simulink model "LKAS_AutoSave_DF_20220408_1006_SW62"  (R2018b)
settings: Solver=FixedStepDiscrete  StartTime=0.0  StopTime=10.0  FixedStep=0.01  RelTol=1e-3
undefined symbols (not defined in the file): LKA_CarWidth, LKA_SampleTime, LKA_StrRatio_C, LKA_Veh2CamL_C, LKA_Veh2CamW_C, LKA_WhlBaseL_C, LL_CompHdAg_C, LL_CompSWA_C, LL_CrvtPrvwT_C, LL_DesDvt_C, LL_DvtComp_C, LL_DvtPrvwT_C, LL_DvtSpdDet_vDvtSpdMin_C, LL_HandsOff_ExitTime, LL_HandsOff_TextTime, LL_HandsOff_WarnTime, LL_HdAgExT_C, LL_HdAgPrvwT_C, LL_LAccMax_C, LL_LAccRMax_C, LL_LDW_EarliestWarnLine_C, LL_LDW_LatestWarnLine_C, LL_LDWS_SUPPRESS_HEADING, LL_LFClb_TFC_FfCtlRatio_C, LL_LFClb_TFC_KdBalance_C, LL_LFClb_TFC_KdMaxSWA_C, LL_LFClb_TFC_KdV1_C, LL_LFClb_TFC_KdV2_C, LL_LFClb_TFC_KdVehSpdLwr_C, LL_LFClb_TFC_KdVehSpdUpr_C, LL_LFClb_TFC_Ki_C, LL_LFClb_TFC_KiMaxSWA_C, LL_LFClb_TFC_Kp_C, LL_LFClb_TFC_KpKlat_C, LL_LFClb_TFC_KpV1_C, LL_LFClb_TFC_KpV2_C, LL_LFClb_TFC_KpVehSpdLwr_C, LL_LFClb_TFC_KpVehSpdUpr_C, LL_LFClb_TFC_PrvwT_C, LL_LKA_EarliestWarnLine_C, LL_LKA_LatestWarnLine_C, LL_LKAExPrcs_ExitC0Dvt, LL_LKAExPrcs_ExitC0Swt, LL_LKAExPrcs_tiExitDelayTime3, LL_LKAExPrcs_tiExitTime1, LL_LKAExPrcs_tiExitTime2, LL_LKAExPrcs_tiExitTime3, LL_LKAS_OUT_OF_CONTROL_LAT_VEL, LL_LKAS_OUT_OF_CONTROL_TTLC, LL_LKASWASyn_M0, LL_LKASWASyn_M1, LL_LKASWASyn_M2, LL_LKASWASyn_M3D, LL_LKASWASyn_M3K_DT, LL_LKASWASyn_M3K_MSD, LL_LKASWASyn_M4K, LL_LKASWASyn_SWAaddMax, LL_LKASWASyn_T2, LL_LKASWASyn_tiTrqSwaRtTime, LL_LKASWASyn_tiTrqSwaTime ... (+47)
libraries: simulink x234, canmsglib x6, dspstat3 x3, simulink_extras x1
(part 1 of 16)
settings Model: Creator=hejr  LastModifiedBy=hejr
settings OptimizationCC: BlockReduction=off  DefaultParameterBehavior=Inlined  UseDivisionForNetSlopeComputation=on  UseFloatMulNetSlope=on  DefaultUnderspecifiedDataType=single  UseSpecifiedMinMax=on  InlineInvariantSignals=on  PassReuseOutputArgsAs=Individual arguments  ZeroExternalMemoryAtStartup=off  ZeroInternalMemoryAtStartup=off  NoFixptDivByZeroProtection=on  EfficientFloat2IntCast=on  LifeSpan=inf  OptimizeBlockOrder=speed  DifferentSizesBufferReuse=on
settings DebuggingCC: SignalInfNanChecking=error  ReadBeforeWriteMsg=EnableAllAsError  WriteAfterWriteMsg=EnableAllAsError  WriteAfterReadMsg=EnableAllAsError  IntegerOverflowMsg=error  ParameterTunabilityLossMsg=error  UniqueDataStoreMsg=error  AssertControl=DisableAll  NonBusSignalsTreatedAsBus=error  SFInvalidInputDataAccessInChartInitDiag=error  SFTransitionOutsideNaturalParentDiag=error  SFUnreachableExecutionPathDiag=error  SFUndirectedBroadcastEventsDiag=error  IntegerSaturationMsg=error
settings HardwareCC: ProdLongLongMode=on
settings ModelReferenceCC: UpdateModelReferenceTargets=IfOutOfDate
settings SFSimCC: SFSimEcho=off  CompileTimeRecursionLimit=0  EnableRuntimeRecursion=off  MATLABDynamicMemAlloc=off
settings RTWCC: SystemTargetFile=autosar.tlc  GenCodeOnly=on  TemplateMakefile=ert_default_tmf  Description=AUTOSAR  GenerateReport=on  BuildConfiguration=Faster Runs  IncludeHyperlinkInReport=on  LaunchReport=on  GenerateTraceInfo=on  GenerateTraceReport=on  GenerateTraceReportSl=on  GenerateTraceReportSf=on  GenerateTraceReportEml=on  GenerateCodeMetricsReport=on  GenerateCodeReplacementReport=on
settings CodeAppCC: ForceParamTrailComments=on  IgnoreCustomStorageClasses=off  OperatorAnnotations=on  SimulinkDataObjDesc=on  SFDataObjDesc=on  MATLABFcnDesc=on  InsertBlockDesc=on  StateflowObjectComments=on  MATLABSourceComments=on  EnableCustomComments=on  ReqsInCode=on
settings STFCustomTargetCC: TargetLangStandard=C99 (ISO)  MultiwordLength=256  ParMdlRefBuildCompliant=on  CompOptLevelCompliant=on  IncludeMdlTerminateFcn=off  CombineOutputUpdateFcns=on  CombineSignalStateStructs=on  SuppressErrorStatus=on  ERTCustomFileBanners=on  SupportNonFinite=off  SupportComplex=off  SupportContinuousTime=off  SupportNonInlinedSFcns=off  RemoveResetFunc=on  ParenthesesLevel=Maximum  CastingMode=Standards  MATLABClassNameForMDSCustomization=Simulink.SoftwareTarget.ERTCustomization  AutosarCompliant=on  UseToolchainInfoCompliant=on  LookupTableObjectStructAxisOrder=2,1,3,4,...  LUTObjectStructOrderEvenSpacing=Size,Table,Breakpoints  SystemTargetFile=autosar.tlc
settings ERTTargetCC: TargetLangStandard=C99 (ISO)  ConcurrentExecutionCompliant=off  IncludeMdlTerminateFcn=off  CombineSignalStateStructs=on  SuppressErrorStatus=on  SupportNonFinite=off  SupportComplex=off  ParenthesesLevel=Maximum  CastingMode=Standards  ModelStepFunctionPrototypeControlCompliant=off  CPPClassGenCompliant=off  AutosarCompliant=on  LookupTableObjectStructAxisOrder=2,1,3,4,...  LUTObjectStructOrderEvenSpacing=Size,Table,Breakpoints  GenerateASAP2=on  InlinedParameterPlacement=NonHierarchical  ERTCustomFileTemplate=example_file_process.tlc  EnableSignedLeftShifts=off  EnableSignedRightShifts=off

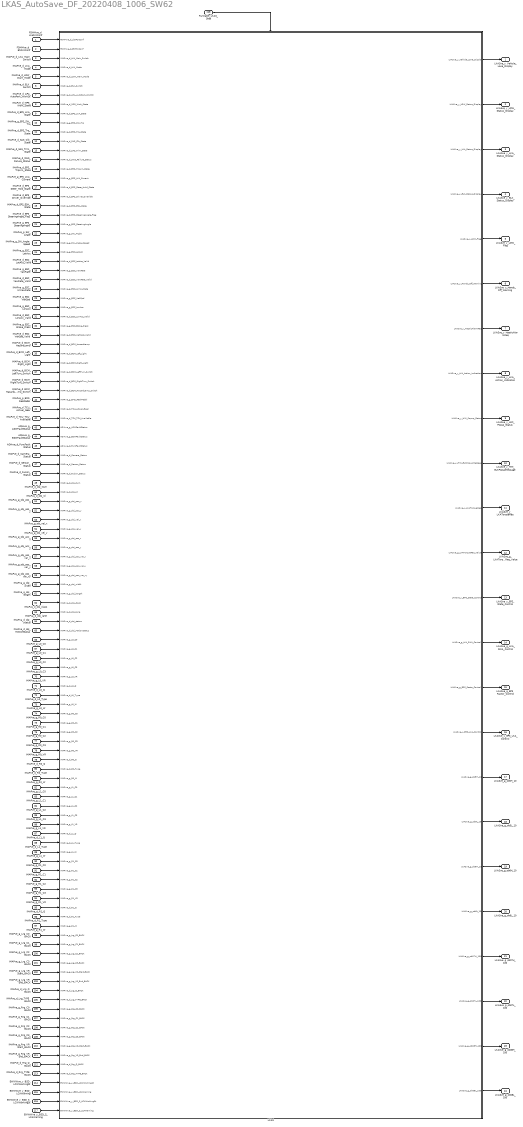
== system LKAS_AutoSave_DF_20220408_1006_SW62 ==
  FDMMve_d_LkaFcnConf : Inport  OutDataTypeStr=UInt16  PortDimensions=1
  FDMMve_d_ElkFcnConf : Inport  Port=2  OutDataTypeStr=UInt16  PortDimensions=1
  IMAPve_d_LKA_Main_Switch : Inport  Port=3  OutDataTypeStr=UInt16  PortDimensions=1
  IMAPve_d_LKA_Mode : Inport  Port=4  OutDataTypeStr=UInt16  PortDimensions=1
  IMAPve_d_LDW_Warn_Mode : Inport  Port=5  OutDataTypeStr=UInt16  PortDimensions=1
  IMAPve_d_ELK_Switch : Inport  Port=6  OutDataTypeStr=UInt16  PortDimensions=1
  IMAPve_d_APA_AutoPark_WorkSt : Inport  Port=7  OutDataTypeStr=UInt16  PortDimensions=1
  IMAPve_d_MP5_Work_State : Inport  Port=8  OutDataTypeStr=UInt16  PortDimensions=1
  IMAPve_d_EPS_LKA_State : Inport  Port=9  OutDataTypeStr=UInt16  PortDimensions=1
  IMAPve_g_EPS_SW_Trq : Inport  Port=10  OutDataTypeStr=T_M_Nm_Float32  PortDimensions=1
  IMAPve_d_EPS_Trq_State : Inport  Port=11  OutDataTypeStr=UInt16  PortDimensions=1
  IMAPve_d_SAS_Clb_State : Inport  Port=12  OutDataTypeStr=UInt16  PortDimensions=1
  IMAPve_d_SAS_Trim_State : Inport  Port=13  OutDataTypeStr=UInt16  PortDimensions=1
  IMAPve_d_SWS_Failure_Status : Inport  Port=14  OutDataTypeStr=UInt16  PortDimensions=1
  IMAPve_d_EPS_TrqLim_State : Inport  Port=15  OutDataTypeStr=UInt16  PortDimensions=1
  IMAPve_g_EPS_LKA_Current : Inport  Port=16  OutDataTypeStr=T_M_Nm_Float32  PortDimensions=1
  IMAPve_d_EPS_Steer_Hold_State : Inport  Port=17  OutDataTypeStr=UInt16  PortDimensions=1
  IMAPve_d_EPS_Driver_Override : Inport  Port=18  OutDataTypeStr=UInt16  PortDimensions=1
  IMAPve_d_EPS_ESA_State : Inport  Port=19  OutDataTypeStr=UInt16  PortDimensions=1
  IMAPve_d_EPS_SteeringAngle_Flag : Inport  Port=20  OutDataTypeStr=UInt16  PortDimensions=1
  IMAPve_g_EPS_SteeringAngle : Inport  Port=21  OutDataTypeStr=T_M_Nm_Float32  PortDimensions=1
  IMAPve_g_SW_Angle : Inport  Port=22  OutDataTypeStr=T_M_Nm_Float32  PortDimensions=1
  IMAPve_g_SW_Angle_Speed : Inport  Port=23  OutDataTypeStr=T_M_Nm_Float32  PortDimensions=1
  IMAPve_g_ESC_LatAcc : Inport  Port=24  OutDataTypeStr=T_M_Nm_Float32  PortDimensions=1
  IMAPve_d_ESC_LatAcc_Valid : Inport  Port=25  OutDataTypeStr=UInt16  PortDimensions=1
  IMAPve_g_ESC_YawRate : Inport  Port=26  OutDataTypeStr=T_M_Nm_Float32  PortDimensions=1
  IMAPve_d_ESC_YawRate_Valid : Inport  Port=27  OutDataTypeStr=UInt16  PortDimensions=1
  IMAPve_g_ESC_UnYawRate : Inport  Port=28  OutDataTypeStr=T_M_Nm_Float32  PortDimensions=1
  IMAPve_g_ESC_VehSpd : Inport  Port=29  OutDataTypeStr=T_M_Nm_Float32  PortDimensions=1
  IMAPve_g_ESC_LonAcc : Inport  Port=30  OutDataTypeStr=T_M_Nm_Float32  PortDimensions=1
  IMAPve_d_ESC_LonAcc_Valid : Inport  Port=31  OutDataTypeStr=UInt16  PortDimensions=1
  IMAPve_g_ESC_Brake_Press : Inport  Port=32  OutDataTypeStr=T_M_Nm_Float32  PortDimensions=1
  IMAPve_d_ESC_VehSpd_Valid : Inport  Port=33  OutDataTypeStr=UInt16  PortDimensions=1
  IMAPve_d_BCM_HazardLamp : Inport  Port=34  OutDataTypeStr=UInt16  PortDimensions=1
  IMAPve_d_BCM_Left_Light : Inport  Port=35  OutDataTypeStr=UInt16  PortDimensions=1
  IMAPve_d_BCM_Right_Light : Inport  Port=36  OutDataTypeStr=UInt16  PortDimensions=1
  IMAPve_d_BCM_LeftTurn_Switch : Inport  Port=37  OutDataTypeStr=UInt16  PortDimensions=1
  IMAPve_d_BCM_RightTurn_Switch : Inport  Port=38  OutDataTypeStr=UInt16  PortDimensions=1
  IMAPve_d_BCM_HazardLamp_Switch : Inport  Port=39  OutDataTypeStr=UInt16  PortDimensions=1
  IMAPve_g_EMS_RealPedal : Inport  Port=40  OutDataTypeStr=T_M_Nm_Float32  PortDimensions=1
  IMAPve_d_TCU_Actual_Gear : Inport  Port=41  OutDataTypeStr=UInt16  PortDimensions=1
  IMAPve_d_TCU_TCU_Available : Inport  Port=42  OutDataTypeStr=UInt16  PortDimensions=1
  ADIAve_g_ASWFaultStatus : Inport  Port=43  OutDataTypeStr=T_M_Nm_Float32  PortDimensions=1
  ADIAve_g_BSWFaultStatus : Inport  Port=44  OutDataTypeStr=T_M_Nm_Float32  PortDimensions=1
  ADIAve_d_FuncFaultStatus : Inport  Port=45  OutDataTypeStr=UInt16  PortDimensions=1
  IMAPve_d_Camera_Status : Inport  Port=46  OutDataTypeStr=UInt16  PortDimensions=1
  IMAPve_d_Sensor_Status : Inport  Port=47  OutDataTypeStr=UInt16  PortDimensions=1
  IMAPve_d_Fusion_Status : Inport  Port=48  OutDataTypeStr=UInt16  PortDimensions=1
  IMAPve_d_obj_Num : Inport  Port=49  OutDataTypeStr=UInt16  PortDimensions=1
  IMAPva_d_obj_id : Inport  Port=50  OutDataTypeStr=UInt16  PortDimensions=40
  IMAPva_g_obj_pos_x : Inport  Port=51  OutDataTypeStr=T_M_Nm_Float32  PortDimensions=40
  IMAPva_g_obj_pos_y : Inport  Port=52  OutDataTypeStr=T_M_Nm_Float32  PortDimensions=40
  IMAPva_g_obj_vel_x : Inport  Port=53  OutDataTypeStr=T_M_Nm_Float32  PortDimensions=40
  IMAPva_g_obj_vel_y : Inport  Port=54  OutDataTypeStr=T_M_Nm_Float32  PortDimensions=40
  IMAPva_g_obj_acc_x : Inport  Port=55  OutDataTypeStr=T_M_Nm_Float32  PortDimensions=40
  IMAPva_g_obj_acc_y : Inport  Port=56  OutDataTypeStr=T_M_Nm_Float32  PortDimensions=40
  IMAPva_g_obj_pos_var_x : Inport  Port=57  OutDataTypeStr=T_M_Nm_Float32  PortDimensions=40
  IMAPva_g_obj_pos_var_y : Inport  Port=58  OutDataTypeStr=T_M_Nm_Float32  PortDimensions=40
  IMAPva_g_obj_pos_var_xy : Inport  Port=59  OutDataTypeStr=T_M_Nm_Float32  PortDimensions=40
  IMAPva_g_obj_width : Inport  Port=60  OutDataTypeStr=T_M_Nm_Float32  PortDimensions=40
  IMAPva_g_obj_length : Inport  Port=61  OutDataTypeStr=T_M_Nm_Float32  PortDimensions=40
  IMAPva_d_obj_class : Inport  Port=62  OutDataTypeStr=UInt16  PortDimensions=40
  IMAPva_d_obj_lane : Inport  Port=63  OutDataTypeStr=UInt16  PortDimensions=40
  IMAPva_d_obj_status : Inport  Port=64  OutDataTypeStr=UInt16  PortDimensions=40
  IMAPva_d_obj_MotionStatus : Inport  Port=65  OutDataTypeStr=UInt16  PortDimensions=40
  IMAPve_g_L0_C0 : Inport  Port=66  OutDataTypeStr=T_M_Nm_Float32  PortDimensions=1
  IMAPve_g_L0_C1 : Inport  Port=67  OutDataTypeStr=T_M_Nm_Float32  PortDimensions=1
  IMAPve_g_L0_C2 : Inport  Port=68  OutDataTypeStr=T_M_Nm_Float32  PortDimensions=1
  IMAPve_g_L0_C3 : Inport  Port=69  OutDataTypeStr=T_M_Nm_Float32  PortDimensions=1
  IMAPve_g_L0_VR : Inport  Port=70  OutDataTypeStr=T_M_Nm_Float32  PortDimensions=1
  IMAPve_d_L0_Q : Inport  Port=71  OutDataTypeStr=UInt16  PortDimensions=1
  IMAPve_d_L0_Type : Inport  Port=72  OutDataTypeStr=UInt16  PortDimensions=1
  IMAPve_g_L0_W : Inport  Port=73  OutDataTypeStr=T_M_Nm_Float32  PortDimensions=1
  IMAPve_g_R0_C0 : Inport  Port=74  OutDataTypeStr=T_M_Nm_Float32  PortDimensions=1
  IMAPve_g_R0_C1 : Inport  Port=75  OutDataTypeStr=T_M_Nm_Float32  PortDimensions=1
  IMAPve_g_R0_C2 : Inport  Port=76  OutDataTypeStr=T_M_Nm_Float32  PortDimensions=1
  IMAPve_g_R0_C3 : Inport  Port=77  OutDataTypeStr=T_M_Nm_Float32  PortDimensions=1
  IMAPve_g_R0_VR : Inport  Port=78  OutDataTypeStr=T_M_Nm_Float32  PortDimensions=1
  IMAPve_d_R0_Q : Inport  Port=79  OutDataTypeStr=UInt16  PortDimensions=1
  IMAPve_d_R0_Type : Inport  Port=80  OutDataTypeStr=UInt16  PortDimensions=1
  IMAPve_g_R0_W : Inport  Port=81  OutDataTypeStr=T_M_Nm_Float32  PortDimensions=1
  IMAPve_g_L1_C0 : Inport  Port=82  OutDataTypeStr=T_M_Nm_Float32  PortDimensions=1
  IMAPve_g_L1_C1 : Inport  Port=83  OutDataTypeStr=T_M_Nm_Float32  PortDimensions=1
  IMAPve_g_L1_C2 : Inport  Port=84  OutDataTypeStr=T_M_Nm_Float32  PortDimensions=1
  IMAPve_g_L1_C3 : Inport  Port=85  OutDataTypeStr=T_M_Nm_Float32  PortDimensions=1
  IMAPve_g_L1_VR : Inport  Port=86  OutDataTypeStr=T_M_Nm_Float32  PortDimensions=1
  IMAPve_d_L1_Q : Inport  Port=87  OutDataTypeStr=UInt16  PortDimensions=1
  IMAPve_d_L1_Type : Inport  Port=88  OutDataTypeStr=UInt16  PortDimensions=1
  IMAPve_g_L1_W : Inport  Port=89  OutDataTypeStr=T_M_Nm_Float32  PortDimensions=1
  IMAPve_g_R1_C0 : Inport  Port=90  OutDataTypeStr=T_M_Nm_Float32  PortDimensions=1
  IMAPve_g_R1_C1 : Inport  Port=91  OutDataTypeStr=T_M_Nm_Float32  PortDimensions=1
  IMAPve_g_R1_C2 : Inport  Port=92  OutDataTypeStr=T_M_Nm_Float32  PortDimensions=1
  IMAPve_g_R1_C3 : Inport  Port=93  OutDataTypeStr=T_M_Nm_Float32  PortDimensions=1
  IMAPve_g_R1_VR : Inport  Port=94  OutDataTypeStr=T_M_Nm_Float32  PortDimensions=1
  IMAPve_d_R1_Q : Inport  Port=95  OutDataTypeStr=UInt16  PortDimensions=1
  IMAPve_d_R1_Type : Inport  Port=96  OutDataTypeStr=UInt16  PortDimensions=1
  IMAPve_g_R1_W : Inport  Port=97  OutDataTypeStr=T_M_Nm_Float32  PortDimensions=1
  IMAPve_g_Lrg_C0_BACK : Inport  Port=98  OutDataTypeStr=T_M_Nm_Float32  PortDimensions=1
  IMAPve_g_Lrg_C1_BACK : Inport  Port=99  OutDataTypeStr=T_M_Nm_Float32  PortDimensions=1
  IMAPve_g_Lrg_C2_BACK : Inport  Port=100  OutDataTypeStr=T_M_Nm_Float32  PortDimensions=1
  IMAPve_g_Lrg_C3_BACK : Inport  Port=101  OutDataTypeStr=T_M_Nm_Float32  PortDimensions=1
  IMAPve_g_Lrg_VR_Start_BACK : Inport  Port=102  OutDataTypeStr=T_M_Nm_Float32  PortDimensions=1
  IMAPve_g_Lrg_VR_End_BACK : Inport  Port=103  OutDataTypeStr=T_M_Nm_Float32  PortDimensions=1
  IMAPve_d_Lrg_Q_BACK : Inport  Port=104  OutDataTypeStr=UInt16  PortDimensions=1
  IMAPve_d_Lrg_TYPE_BACK : Inport  Port=105  OutDataTypeStr=UInt16  PortDimensions=1
  IMAPve_g_Rrg_C0_BACK : Inport  Port=106  OutDataTypeStr=T_M_Nm_Float32  PortDimensions=1
  IMAPve_g_Rrg_C1_BACK : Inport  Port=107  OutDataTypeStr=T_M_Nm_Float32  PortDimensions=1
  IMAPve_g_Rrg_C2_BACK : Inport  Port=108  OutDataTypeStr=T_M_Nm_Float32  PortDimensions=1
  IMAPve_g_Rrg_C3_BACK : Inport  Port=109  OutDataTypeStr=T_M_Nm_Float32  PortDimensions=1
  IMAPve_g_Rrg_VR_Start_BACK : Inport  Port=110  OutDataTypeStr=T_M_Nm_Float32  PortDimensions=1
  IMAPve_g_Rrg_VR_End_BACK : Inport  Port=111  OutDataTypeStr=T_M_Nm_Float32  PortDimensions=1
  IMAPve_d_Rrg_Q_BACK : Inport  Port=112  OutDataTypeStr=UInt16  PortDimensions=1
  IMAPve_d_Rrg_TYPE_BACK : Inport  Port=113  OutDataTypeStr=UInt16  PortDimensions=1
  EWWWve_y_BSD_LCWWorkingSt : Inport  Port=114  OutDataTypeStr=UInt8  PortDimensions=1
  EWWWve_y_BSD_LCAWarning : Inport  Port=115  OutDataTypeStr=UInt8  PortDimensions=1
  EWWWve_y_BSD_S_LCWWorkingSt : Inport  Port=116  OutDataTypeStr=UInt8  PortDimensions=1
  EWWWve_y_BSD_S_LCAWarning : Inport  Port=117  OutDataTypeStr=UInt8  PortDimensions=1
  Runnable_LKAS_Step : Inport  Port=118  SampleTime=0.01  OutputFunctionCall=on
  LKAS : Subsystem  TreatAsAtomicUnit=on
  LKASve_y_Vehicle_Lane_Display : Outport  OutDataTypeStr=UInt8  PortDimensions=1
  LKASve_y_LDW_Status_Display : Outport  Port=2  OutDataTypeStr=UInt8  PortDimensions=1
  LKASve_y_LKA_Status_Display : Outport  Port=3  OutDataTypeStr=UInt8  PortDimensions=1
  LKASve_y_ELK_Status_Display : Outport  Port=4  OutDataTypeStr=UInt8  PortDimensions=1
  LKASve_y_LDW_Flag : Outport  Port=5  OutDataTypeStr=UInt8  PortDimensions=1
  LKASve_y_Hands_Off_Warning : Outport  Port=6  OutDataTypeStr=UInt8  PortDimensions=1
  LKASve_y_HapticAlarmReq : Outport  Port=7  OutDataTypeStr=UInt8  PortDimensions=1
  LKASve_y_LKA_Action_Indication : Outport  Port=8  OutDataTypeStr=UInt8  PortDimensions=1
  LKASve_y_HMI_Popup_Status : Outport  Port=9  OutDataTypeStr=UInt8  PortDimensions=1
  LKASve_y_HMI_ELKPopupMessage : Outport  Port=10  OutDataTypeStr=UInt8  PortDimensions=1
  LKASve_y_LKATorqueReq : Outport  Port=11  OutDataTypeStr=UInt8  PortDimensions=1
  LKASve_g_LKATorqueReq_Value : Outport  Port=12  OutDataTypeStr=T_M_Nm_Float32  PortDimensions=1
  LKASve_y_EPS_State_Control : Outport  Port=13  OutDataTypeStr=UInt8  PortDimensions=1
  LKASve_g_LKA_SWA_Control : Outport  Port=14  OutDataTypeStr=T_M_Nm_Float32  PortDimensions=1
  LKASve_g_EPS_Factor_Control : Outport  Port=15  OutDataTypeStr=T_M_Nm_Float32  PortDimensions=1
  LKASve_y_EPS_LKA_Control : Outport  Port=16  OutDataTypeStr=UInt8  PortDimensions=1
  LKASve_g_ob5H_10 : Outport  Port=17  OutDataTypeStr=UInt32  PortDimensions=1
  LKASve_g_ob5L_10 : Outport  Port=18  OutDataTypeStr=UInt32  PortDimensions=1
  LKASve_g_ob6H_10 : Outport  Port=19  OutDataTypeStr=UInt32  PortDimensions=1
  LKASve_g_ob6L_10 : Outport  Port=20  OutDataTypeStr=UInt32  PortDimensions=1
  LKASve_g_ob07H_100 : Outport  Port=21  OutDataTypeStr=UInt32  PortDimensions=1
  LKASve_g_ob07L_100 : Outport  Port=22  OutDataTypeStr=UInt32  PortDimensions=1
  LKASve_g_ob08H_100 : Outport  Port=23  OutDataTypeStr=UInt32  PortDimensions=1
  LKASve_g_ob08L_100 : Outport  Port=24  OutDataTypeStr=UInt32  PortDimensions=1
  wires:
  FDMMve_d_LkaFcnConf/1 -> LKAS/1(FDMMve_d_LkaFcnConf)
  FDMMve_d_ElkFcnConf/1 -> LKAS/2(FDMMve_d_ElkFcnConf)
  IMAPve_d_LKA_Main_Switch/1 -> LKAS/3(IMAPve_d_LKA_Main_Switch)
  IMAPve_d_LKA_Mode/1 -> LKAS/4(IMAPve_d_LKA_Mode)
  IMAPve_d_LDW_Warn_Mode/1 -> LKAS/5(IMAPve_d_LDW_Warn_Mode)
  IMAPve_d_ELK_Switch/1 -> LKAS/6(IMAPve_d_ELK_Switch)
  IMAPve_d_APA_AutoPark_WorkSt/1 -> LKAS/7(IMAPve_d_APA_AutoPark_WorkSt)
  IMAPve_d_MP5_Work_State/1 -> LKAS/8(IMAPve_d_MP5_Work_State)
  IMAPve_d_EPS_LKA_State/1 -> LKAS/9(IMAPve_d_EPS_LKA_State)
  IMAPve_g_EPS_SW_Trq/1 -> LKAS/10(IMAPve_g_EPS_SW_Trq)
  IMAPve_d_EPS_Trq_State/1 -> LKAS/11(IMAPve_d_EPS_Trq_State)
  IMAPve_d_SAS_Clb_State/1 -> LKAS/12(IMAPve_d_SAS_Clb_State)
  IMAPve_d_SAS_Trim_State/1 -> LKAS/13(IMAPve_d_SAS_Trim_State)
  IMAPve_d_SWS_Failure_Status/1 -> LKAS/14(IMAPve_d_SWS_Failure_Status)
  IMAPve_d_EPS_TrqLim_State/1 -> LKAS/15(IMAPve_d_EPS_TrqLim_State)
  IMAPve_g_EPS_LKA_Current/1 -> LKAS/16(IMAPve_g_EPS_LKA_Current)
  IMAPve_d_EPS_Steer_Hold_State/1 -> LKAS/17(IMAPve_d_EPS_Steer_Hold_State)
  IMAPve_d_EPS_Driver_Override/1 -> LKAS/18(IMAPve_d_EPS_Driver_Override)
  IMAPve_d_EPS_ESA_State/1 -> LKAS/19(IMAPve_d_EPS_ESA_State)
  IMAPve_d_EPS_SteeringAngle_Flag/1 -> LKAS/20(IMAPve_d_EPS_SteeringAngle_Flag)
  IMAPve_g_EPS_SteeringAngle/1 -> LKAS/21(IMAPve_g_EPS_SteeringAngle)
  IMAPve_g_SW_Angle/1 -> LKAS/22(IMAPve_g_SW_Angle)
  IMAPve_g_SW_Angle_Speed/1 -> LKAS/23(IMAPve_g_SW_Angle_Speed)
  IMAPve_g_ESC_LatAcc/1 -> LKAS/24(IMAPve_g_ESC_LatAcc)
  IMAPve_d_ESC_LatAcc_Valid/1 -> LKAS/25(IMAPve_d_ESC_LatAcc_Valid)
  IMAPve_g_ESC_YawRate/1 -> LKAS/26(IMAPve_g_ESC_YawRate)
  IMAPve_d_ESC_YawRate_Valid/1 -> LKAS/27(IMAPve_d_ESC_YawRate_Valid)
  IMAPve_g_ESC_UnYawRate/1 -> LKAS/28(IMAPve_g_ESC_UnYawRate)
  IMAPve_g_ESC_VehSpd/1 -> LKAS/29(IMAPve_g_ESC_VehSpd)
  IMAPve_g_ESC_LonAcc/1 -> LKAS/30(IMAPve_g_ESC_LonAcc)
  IMAPve_d_ESC_LonAcc_Valid/1 -> LKAS/31(IMAPve_d_ESC_LonAcc_Valid)
  IMAPve_g_ESC_Brake_Press/1 -> LKAS/32(IMAPve_g_ESC_Brake_Press)
  IMAPve_d_ESC_VehSpd_Valid/1 -> LKAS/33(IMAPve_d_ESC_VehSpd_Valid)
  IMAPve_d_BCM_HazardLamp/1 -> LKAS/34(IMAPve_d_BCM_HazardLamp)
  IMAPve_d_BCM_Left_Light/1 -> LKAS/35(IMAPve_d_BCM_Left_Light)
  IMAPve_d_BCM_Right_Light/1 -> LKAS/36(IMAPve_d_BCM_Right_Light)
  IMAPve_d_BCM_LeftTurn_Switch/1 -> LKAS/37(IMAPve_d_BCM_LeftTurn_Switch)
  IMAPve_d_BCM_RightTurn_Switch/1 -> LKAS/38(IMAPve_d_BCM_RightTurn_Switch)
  IMAPve_d_BCM_HazardLamp_Switch/1 -> LKAS/39(IMAPve_d_BCM_HazardLamp_Switch)
  IMAPve_g_EMS_RealPedal/1 -> LKAS/40(IMAPve_g_EMS_RealPedal)
  IMAPve_d_TCU_Actual_Gear/1 -> LKAS/41(IMAPve_d_TCU_Actual_Gear)
  IMAPve_d_TCU_TCU_Available/1 -> LKAS/42(IMAPve_d_TCU_TCU_Available)
  ADIAve_g_ASWFaultStatus/1 -> LKAS/43(ADIAve_g_ASWFaultStatus)
  ADIAve_g_BSWFaultStatus/1 -> LKAS/44(ADIAve_g_BSWFaultStatus)
  ADIAve_d_FuncFaultStatus/1 -> LKAS/45(ADIAve_d_FuncFaultStatus)
  IMAPve_d_Camera_Status/1 -> LKAS/46(IMAPve_d_Camera_Status)
  IMAPve_d_Sensor_Status/1 -> LKAS/47(IMAPve_d_Sensor_Status)
  IMAPve_d_Fusion_Status/1 -> LKAS/48(IMAPve_d_Fusion_Status)
  IMAPve_d_obj_Num/1 -> LKAS/49(IMAPve_d_obj_Num)
  IMAPva_d_obj_id/1 -> LKAS/50(IMAPva_d_obj_id)
  IMAPva_g_obj_pos_x/1 -> LKAS/51(IMAPva_g_obj_pos_x)
  IMAPva_g_obj_pos_y/1 -> LKAS/52(IMAPva_g_obj_pos_y)
  IMAPva_g_obj_vel_x/1 -> LKAS/53(IMAPva_g_obj_vel_x)
  IMAPva_g_obj_vel_y/1 -> LKAS/54(IMAPva_g_obj_vel_y)
  IMAPva_g_obj_acc_x/1 -> LKAS/55(IMAPva_g_obj_acc_x)
  IMAPva_g_obj_acc_y/1 -> LKAS/56(IMAPva_g_obj_acc_y)
  IMAPva_g_obj_pos_var_x/1 -> LKAS/57(IMAPva_g_obj_pos_var_x)
  IMAPva_g_obj_pos_var_y/1 -> LKAS/58(IMAPva_g_obj_pos_var_y)
  IMAPva_g_obj_pos_var_xy/1 -> LKAS/59(IMAPva_g_obj_pos_var_xy)
  IMAPva_g_obj_width/1 -> LKAS/60(IMAPva_g_obj_width)
  IMAPva_g_obj_length/1 -> LKAS/61(IMAPva_g_obj_length)
  IMAPva_d_obj_class/1 -> LKAS/62(IMAPva_d_obj_class)
  IMAPva_d_obj_lane/1 -> LKAS/63(IMAPva_d_obj_lane)
  IMAPva_d_obj_status/1 -> LKAS/64(IMAPva_d_obj_status)
  IMAPva_d_obj_MotionStatus/1 -> LKAS/65(IMAPva_d_obj_MotionStatus)
  IMAPve_g_L0_C0/1 -> LKAS/66(IMAPve_g_L0_C0)
  IMAPve_g_L0_C1/1 -> LKAS/67(IMAPve_g_L0_C1)
  IMAPve_g_L0_C2/1 -> LKAS/68(IMAPve_g_L0_C2)
  IMAPve_g_L0_C3/1 -> LKAS/69(IMAPve_g_L0_C3)
  IMAPve_g_L0_VR/1 -> LKAS/70(IMAPve_g_L0_VR)
  IMAPve_d_L0_Q/1 -> LKAS/71(IMAPve_d_L0_Q)
  IMAPve_d_L0_Type/1 -> LKAS/72(IMAPve_d_L0_Type)
  IMAPve_g_L0_W/1 -> LKAS/73(IMAPve_g_L0_W)
  IMAPve_g_R0_C0/1 -> LKAS/74(IMAPve_g_R0_C0)
  IMAPve_g_R0_C1/1 -> LKAS/75(IMAPve_g_R0_C1)
  IMAPve_g_R0_C2/1 -> LKAS/76(IMAPve_g_R0_C2)
  IMAPve_g_R0_C3/1 -> LKAS/77(IMAPve_g_R0_C3)
  IMAPve_g_R0_VR/1 -> LKAS/78(IMAPve_g_R0_VR)
  IMAPve_d_R0_Q/1 -> LKAS/79(IMAPve_d_R0_Q)
  IMAPve_d_R0_Type/1 -> LKAS/80(IMAPve_d_R0_Type)
  IMAPve_g_R0_W/1 -> LKAS/81(IMAPve_g_R0_W)
  IMAPve_g_L1_C0/1 -> LKAS/82(IMAPve_g_L1_C0)
  IMAPve_g_L1_C1/1 -> LKAS/83(IMAPve_g_L1_C1)
  IMAPve_g_L1_C2/1 -> LKAS/84(IMAPve_g_L1_C2)
  IMAPve_g_L1_C3/1 -> LKAS/85(IMAPve_g_L1_C3)
  IMAPve_g_L1_VR/1 -> LKAS/86(IMAPve_g_L1_VR)
  IMAPve_d_L1_Q/1 -> LKAS/87(IMAPve_d_L1_Q)
  IMAPve_d_L1_Type/1 -> LKAS/88(IMAPve_d_L1_Type)
  IMAPve_g_L1_W/1 -> LKAS/89(IMAPve_g_L1_W)
  IMAPve_g_R1_C0/1 -> LKAS/90(IMAPve_g_R1_C0)
  IMAPve_g_R1_C1/1 -> LKAS/91(IMAPve_g_R1_C1)
  IMAPve_g_R1_C2/1 -> LKAS/92(IMAPve_g_R1_C2)
  IMAPve_g_R1_C3/1 -> LKAS/93(IMAPve_g_R1_C3)
  IMAPve_g_R1_VR/1 -> LKAS/94(IMAPve_g_R1_VR)
  IMAPve_d_R1_Q/1 -> LKAS/95(IMAPve_d_R1_Q)
  IMAPve_d_R1_Type/1 -> LKAS/96(IMAPve_d_R1_Type)
  IMAPve_g_R1_W/1 -> LKAS/97(IMAPve_g_R1_W)
  IMAPve_g_Lrg_C0_BACK/1 -> LKAS/98(IMAPve_g_Lrg_C0_BACK)
  IMAPve_g_Lrg_C1_BACK/1 -> LKAS/99(IMAPve_g_Lrg_C1_BACK)
  IMAPve_g_Lrg_C2_BACK/1 -> LKAS/100(IMAPve_g_Lrg_C2_BACK)
  IMAPve_g_Lrg_C3_BACK/1 -> LKAS/101(IMAPve_g_Lrg_C3_BACK)
  IMAPve_g_Lrg_VR_Start_BACK/1 -> LKAS/102(IMAPve_g_Lrg_VR_Start_BACK)
  IMAPve_g_Lrg_VR_End_BACK/1 -> LKAS/103(IMAPve_g_Lrg_VR_End_BACK)
  IMAPve_d_Lrg_Q_BACK/1 -> LKAS/104(IMAPve_d_Lrg_Q_BACK)
  IMAPve_d_Lrg_TYPE_BACK/1 -> LKAS/105(IMAPve_d_Lrg_TYPE_BACK)
  IMAPve_g_Rrg_C0_BACK/1 -> LKAS/106(IMAPve_g_Rrg_C0_BACK)
  IMAPve_g_Rrg_C1_BACK/1 -> LKAS/107(IMAPve_g_Rrg_C1_BACK)
  IMAPve_g_Rrg_C2_BACK/1 -> LKAS/108(IMAPve_g_Rrg_C2_BACK)
  IMAPve_g_Rrg_C3_BACK/1 -> LKAS/109(IMAPve_g_Rrg_C3_BACK)
  IMAPve_g_Rrg_VR_Start_BACK/1 -> LKAS/110(IMAPve_g_Rrg_VR_Start_BACK)
  IMAPve_g_Rrg_VR_End_BACK/1 -> LKAS/111(IMAPve_g_Rrg_VR_End_BACK)
  IMAPve_d_Rrg_Q_BACK/1 -> LKAS/112(IMAPve_d_Rrg_Q_BACK)
  IMAPve_d_Rrg_TYPE_BACK/1 -> LKAS/113(IMAPve_d_Rrg_TYPE_BACK)
  EWWWve_y_BSD_LCWWorkingSt/1 -> LKAS/114(EWWWve_y_BSD_LCWWorkingSt)
  EWWWve_y_BSD_LCAWarning/1 -> LKAS/115(EWWWve_y_BSD_LCAWarning)
  EWWWve_y_BSD_S_LCWWorkingSt/1 -> LKAS/116(EWWWve_y_BSD_S_LCWWorkingSt)
  EWWWve_y_BSD_S_LCAWarning/1 -> LKAS/117(EWWWve_y_BSD_S_LCAWarning)
  Runnable_LKAS_Step/1 -> LKAS/Trigger
  LKAS/1(LKASve_y_Vehicle_Lane_Display) -> LKASve_y_Vehicle_Lane_Display/1
  LKAS/2(LKASve_y_LDW_Status_Display) -> LKASve_y_LDW_Status_Display/1
  LKAS/3(LKASve_y_LKA_Status_Display) -> LKASve_y_LKA_Status_Display/1
  LKAS/4(LKASve_y_ELK_Status_Display) -> LKASve_y_ELK_Status_Display/1
  LKAS/5(LKASve_y_LDW_Flag) -> LKASve_y_LDW_Flag/1
  LKAS/6(LKASve_y_Hands_Off_Warning) -> LKASve_y_Hands_Off_Warning/1
  LKAS/7(LKASve_y_HapticAlarmReq) -> LKASve_y_HapticAlarmReq/1
  LKAS/8(LKASve_y_LKA_Action_Indication) -> LKASve_y_LKA_Action_Indication/1
  LKAS/9(LKASve_y_HMI_Popup_Status) -> LKASve_y_HMI_Popup_Status/1
  LKAS/10(LKASve_y_HMI_ELKPopupMessage) -> LKASve_y_HMI_ELKPopupMessage/1
  LKAS/11(LKASve_y_LKATorqueReq) -> LKASve_y_LKATorqueReq/1
  LKAS/12(LKASve_g_LKATorqueReq_Value) -> LKASve_g_LKATorqueReq_Value/1
  LKAS/13(LKASve_y_EPS_State_Control) -> LKASve_y_EPS_State_Control/1
  LKAS/14(LKASve_g_LKA_SWA_Control) -> LKASve_g_LKA_SWA_Control/1
  LKAS/15(LKASve_g_EPS_Factor_Control) -> LKASve_g_EPS_Factor_Control/1
  LKAS/16(LKASve_y_EPS_LKA_Control) -> LKASve_y_EPS_LKA_Control/1
  LKAS/17(LKASve_g_ob5H_10) -> LKASve_g_ob5H_10/1
  LKAS/18(LKASve_g_ob5L_10) -> LKASve_g_ob5L_10/1
  LKAS/19(LKASve_g_ob6H_10) -> LKASve_g_ob6H_10/1
  LKAS/20(LKASve_g_ob6L_10) -> LKASve_g_ob6L_10/1
  LKAS/21(LKASve_g_ob07H_100) -> LKASve_g_ob07H_100/1
  LKAS/22(LKASve_g_ob07L_100) -> LKASve_g_ob07L_100/1
  LKAS/23(LKASve_g_ob08H_100) -> LKASve_g_ob08H_100/1
  LKAS/24(LKASve_g_ob08L_100) -> LKASve_g_ob08L_100/1
